simulink model "pc_data_rx"  (R2022a)
settings: Solver=VariableStepAuto  StartTime=0.0  StopTime=inf  RelTol=1e-3
libraries: instrumentseriallib x2, embeddedblockslib x1
settings Model: Creator=EEED Stores 381  LastModifiedBy=EEED Stores 381

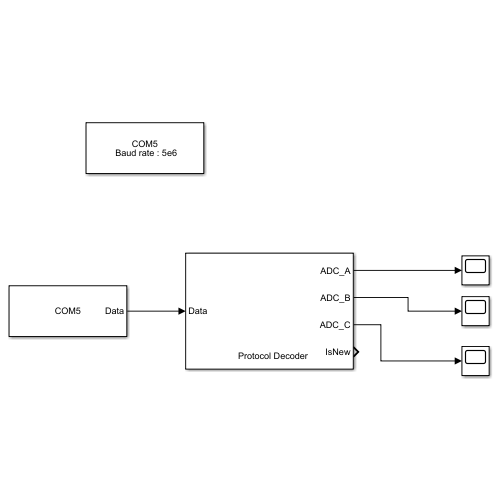
[thumbnail: Simulink's stored preview of the top-level diagram]
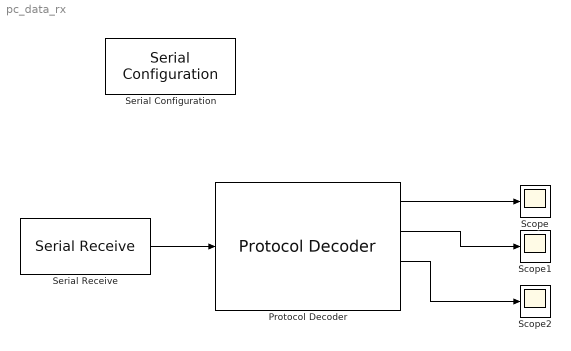
== system pc_data_rx ==
  Protocol Decoder : embeddedblockslib/Protocol Decoder  IsParseCSV=off  Header='S'  FieldTable={ 'ADC_A', '1', 'uint16', 'Little endian'; 'ADC_B', '1', 'uint16', 'Little endian'; 'ADC_C', '1', 'uint16', 'Little endian' }  IsVariableSizeLastField=off  MaxVariableSizeFieldLength=[]  IsChecksumRequired=off  ChecksumAlgorithm=XOR of bytes  ChecksumSize=[]  TerminatorOption=<none>  CustomTerminatorVal=[]  IsInputLengthAvailable=off
      settings: SourceProductBaseCode=ARDUINO,TIC2000
  Scope : Scope
  Scope1 : Scope
  Scope2 : Scope
  Serial Configuration : instrumentseriallib/Serial Configuration  Priority=-200000  PortSel=COM5  Port=COM5  ComPort=COM5  BaudRate=5e6  DataBits=8  Parity=none  StopBits=1  ByteOrder=little-endian  FlowControl=none  Timeout=10  SimulateUsing=Interpreted execution  BlockInModel=on  aMode=1
  Serial Receive : instrumentseriallib/Serial Receive  Priority=1  PortSel=COM5  Port=COM5  ComPort=COM5  DataType=uint8  SaveDataType=uint8  ToggleHeader=off  Header=[]  ToggleTerminator=off  Terminator=<none>  CustomTerminator=[]  InputFormat=Column major  ToggleDataSize=on  DataSize=2  EnableBlockingMode=on  ActionDataUnavailable=Output last received value  ActionWhenDataUnavailable=Output last received value  CustomValue=0  SampleTime=0.001  SimulateUsing=Interpreted execution  BlockInModel=on  aMode=1
      settings: SourceProductBaseCode=OT,IC,MT
  wires:
  Serial Receive/1 -> Protocol Decoder/1
  Protocol Decoder/1 -> Scope/1
  Protocol Decoder/2 -> Scope1/1
  Protocol Decoder/3 -> Scope2/1
